simulink model "obiekt1"  (R2016b)
settings: Solver=ode45  StartTime=0.0  StopTime=100  RelTol=1e-3  EnableMultiTasking=on
values from neighbouring files (symbols this model uses):
  A1 = A.'    [z1.m]
  B1 = C.'    [z1.m]
settings Model: Creator=Agnieszka i Kamilka  LastModifiedBy=kamil
settings DataIOCC: LimitDataPoints=on  SaveFormat=Array  SignalLoggingSaveFormat=ModelDataLogs
settings OptimizationCC: ExpressionDepthLimit=2147483647  LifeSpan=inf
settings DebuggingCC: UnderspecifiedInitializationDetection=Classic  MergeDetectMultiDrivingBlocksExec=none  SolverPrmCheckMsg=warning  FcnCallInpInsideContextMsg=warning  StateNameClashWarn=warning  SFUnexpectedBacktrackingDiag=warning  SFNoUnconditionalDefaultTransitionDiag=warning  SFExecutionAtInitializationDiag=none
settings HardwareCC: ProdBitPerPointer=32  ProdBitPerSizeT=32  ProdBitPerPtrDiffT=32  ProdLargestAtomicFloat=None  ProdIntDivRoundTo=Undefined  ProdEndianess=Unspecified  ProdWordSize=32  ProdHWDeviceType=32-bit Generic
settings ModelReferenceCC: PropagateSignalLabelsOutOfModel=off
settings GRTTargetCC: TargetLangStandard=C89/C90 (ANSI)  GeneratePreprocessorConditionals=Disable all  CombineOutputUpdateFcns=off  GRTInterface=on
settings ConfigComp: CovMetricSettings=dw  CovHtmlReporting=on  CovSaveCumulativeToWorkspaceVar=on  CovSaveSingleToWorkspaceVar=on  CovExternalEMLEnable=off

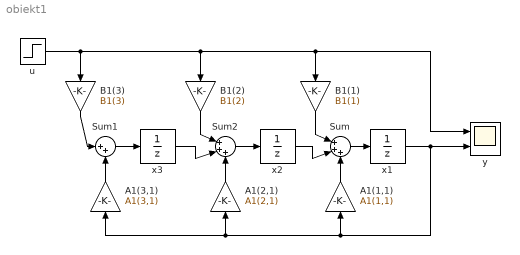
== system obiekt1 ==
  A1(1,1) : Gain  Gain=A1(1,1)
  A1(2,1) : Gain  Gain=A1(2,1)
  A1(3,1) : Gain  Gain=A1(3,1)
  B1(1) : Gain  Gain=B1(1)
  B1(2) : Gain  Gain=B1(2)
  B1(3) : Gain  Gain=B1(3)
  Sum : Sum  Inputs=|+++
  Sum1 : Sum  Inputs=|++
  Sum2 : Sum  Inputs=|+++
  u : Step  After=0.1  SampleTime=0
  x1 : UnitDelay  SampleTime=-1
  x2 : UnitDelay  SampleTime=-1
  x3 : UnitDelay  SampleTime=-1
  y : Scope  NumInputPorts=2
  wires:
  B1(3)/1 -> Sum1/1
  u/1 -> y/1, B1(1)/1, B1(2)/1, B1(3)/1
  Sum1/1 -> x3/1
  x1/1 -> y/2, A1(3,1)/1, A1(2,1)/1, A1(1,1)/1
  A1(1,1)/1 -> Sum/3
  A1(2,1)/1 -> Sum2/3
  A1(3,1)/1 -> Sum1/2
  Sum/1 -> x1/1
  x2/1 -> Sum/2
  Sum2/1 -> x2/1
  x3/1 -> Sum2/2
  B1(1)/1 -> Sum/1
  B1(2)/1 -> Sum2/1
